simulink model "kadai2"  (R2019b)
settings: Solver=VariableStepAuto  StartTime=0.0  StopTime=10.0  RelTol=1e-3
values from neighbouring files (symbols this model uses):
  D = 1    [ex01.m]
  J = 1    [ex01.m]
  Kt = 1    [ex01.m]
settings Model: Creator=ryoga  LastModifiedBy=ryoga

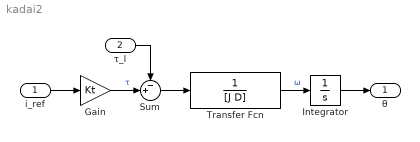
== system kadai2 ==
  i_ref : Inport
  τ_l : Inport  Port=2
  Gain : Gain  Gain=Kt
  Integrator : Integrator
  Sum : Sum  Inputs=-+|
  Transfer Fcn : TransferFcn  Denominator=[J D]
  θ : Outport
  wires:
  Sum/1 -> Transfer Fcn/1
  Gain/1 -> Sum/2  "τ"
  i_ref/1 -> Gain/1
  τ_l/1 -> Sum/1
  Transfer Fcn/1 -> Integrator/1  "ω"
  Integrator/1 -> θ/1
